simulink model "problem5"  (R2020b)
settings: Solver=VariableStepAuto  StartTime=0.0  StopTime=10  RelTol=1e-3
model workspace (MAT data in the model file):
  C = Simulink.Parameter
  C.Value = 0.1
  C.DataType = 'auto'
  C.Dimensions = [1 1]
  R = Simulink.Parameter
  R.Value = 10
  R.DataType = 'auto'
  R.Dimensions = [1 1]
settings Model: Creator=admin  LastModifiedBy=admin

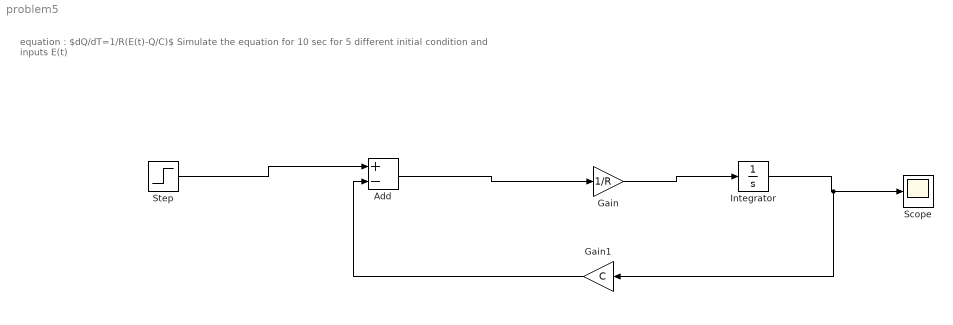
== system problem5 ==
  note: equation : $dQ/dT=1/R(E(t)-Q/C)$
      | Simulate the equation for 10 sec for 5 different initial condition and inputs E(t)
  Add : Sum  Inputs=+-
  Gain : Gain  Gain=1/R
  Gain1 : Gain  Gain=C
  Integrator : Integrator
  Scope : Scope
  Step : Step  Before=4  SampleTime=0
  wires:
  Add/1 -> Gain/1
  Gain/1 -> Integrator/1
  Integrator/1 -> Gain1/1, Scope/1
  Step/1 -> Add/1
  Gain1/1 -> Add/2
